simulink model "saturate_int_test_tmp"  (Simulink 8.3)
settings: Solver=VariableStepDiscrete  StartTime=0.0  StopTime=10.0  RelTol=1e-3
settings Model: Creator=arnaud  LastModifiedBy=hbourbou  CovSFcnEnable=on
settings DataIOCC: SaveFormat=Structure
settings OptimizationCC: ExpressionDepthLimit=2147483647
settings DebuggingCC: FcnCallInpInsideContextMsg=EnableAllAsWarning  FrameProcessingCompatibilityMsg=error  StrictBusMsg=Warning
settings GRTTargetCC: GeneratePreprocessorConditionals=Use local settings

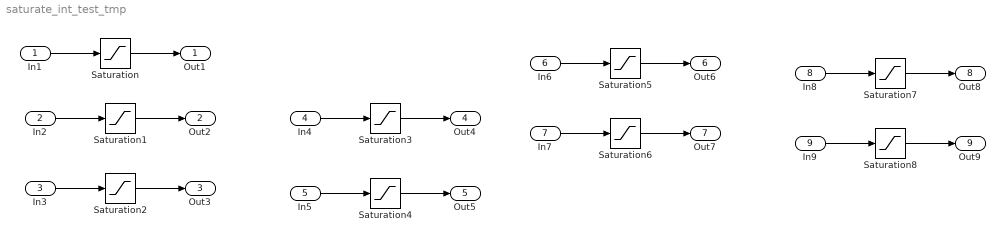
== system saturate_int_test_tmp ==
  In1 : Inport  OutDataTypeStr=double
  In2 : Inport  Port=2  OutDataTypeStr=double  PortDimensions=3
  In3 : Inport  Port=3  OutDataTypeStr=double  PortDimensions=[2 3]
  In4 : Inport  Port=4  OutDataTypeStr=double  PortDimensions=3
  In5 : Inport  Port=5  OutDataTypeStr=double  PortDimensions=[2 3]
  In6 : Inport  Port=6  OutDataTypeStr=double
  In7 : Inport  Port=7  OutDataTypeStr=double
  In8 : Inport  Port=8  OutDataTypeStr=double
  In9 : Inport  Port=9  OutDataTypeStr=double
  Saturation : Saturate  UpperLimit=0.6
  Saturation1 : Saturate  UpperLimit=0.4  RndMeth=Ceiling
  Saturation2 : Saturate  UpperLimit=0.6  RndMeth=Nearest
  Saturation3 : Saturate  UpperLimit=[0.4 0.6 0.7]  LowerLimit=[-0.5 -0.6 -0.7]  RndMeth=Zero
  Saturation4 : Saturate  UpperLimit=[0.5 0.6 0.7; 1.5 1.6 1.7]  LowerLimit=[-0.5 -0.6 -0.7; -1.5 -1.6 -1.7]  RndMeth=Zero
  Saturation5 : Saturate  UpperLimit=[2 3 4]  LowerLimit=[-2 -3 -4]
  Saturation6 : Saturate  UpperLimit=[2 3 4; 5 6 7]  LowerLimit=[-2 -3 -4; -5 -6 -7]
  Saturation7 : Saturate  UpperLimit=2  LowerLimit=[-2 -3 -4]
  Saturation8 : Saturate  UpperLimit=[2 3 4; 5 6 7]  LowerLimit=-2
  Out1 : Outport
  Out2 : Outport  Port=2
  Out3 : Outport  Port=3
  Out4 : Outport  Port=4
  Out5 : Outport  Port=5
  Out6 : Outport  Port=6
  Out7 : Outport  Port=7
  Out8 : Outport  Port=8
  Out9 : Outport  Port=9
  wires:
  In1/1 -> Saturation/1
  Saturation/1 -> Out1/1
  In2/1 -> Saturation1/1
  Saturation1/1 -> Out2/1
  In3/1 -> Saturation2/1
  Saturation2/1 -> Out3/1
  In4/1 -> Saturation3/1
  Saturation3/1 -> Out4/1
  In5/1 -> Saturation4/1
  Saturation4/1 -> Out5/1
  In6/1 -> Saturation5/1
  Saturation5/1 -> Out6/1
  In7/1 -> Saturation6/1
  Saturation6/1 -> Out7/1
  In8/1 -> Saturation7/1
  Saturation7/1 -> Out8/1
  In9/1 -> Saturation8/1
  Saturation8/1 -> Out9/1
